simulink model "SG__DMA_test"  (R2022b)
settings: Solver=FixedStepAuto  StartTime=0.0  StopTime=2  FixedStep=50e-6  RelTol=1e-3  EnableMultiTasking=on
undefined symbols (not defined in the file or in its folder): Ended, Single
libraries: speedgoatlib_IO104 x3, speedgoatlib_IO135 x3, dspsrcs4 x2, speedgoatlib_interrupt x1
Description:
  | IO135 - DMA Loopback
settings Model: sg_rtwmakecfg_data=_sglibc_  ModifiedByFormat=Speedgoat  SimulationMode=external  PauseTimes=0  ExtModeTrigDuration=100000  Creator=Speedgoat  LastModifiedBy=Speedgoat
settings SolverCC: ConcurrentTasks=on  AlgebraicLoopSolver=TrustRegion  PositivePriorityOrder=on  AutoInsertRateTranBlk=on  InsertRTBMode=Never (minimum delay)
settings DataIOCC: SaveFormat=StructureWithTime  ReturnWorkspaceOutputs=off
settings OptimizationCC: BlockReduction=off  OptimizeBlockIOStorage=off  BufferReuse=off  ReuseModelBlockBuffer=on  GlobalBufferReuse=off  ExpressionFolding=off  LocalBlockOutputs=off
settings DebuggingCC: TasksWithSamePriorityMsg=none  UnconnectedInputMsg=warning  UnconnectedOutputMsg=warning  UnconnectedLineMsg=warning  SFExecutionAtInitializationDiag=none  ArithmeticOperatorsInVariantConditions=warning
settings HardwareCC: ProdBitPerLong=64  ProdLongLongMode=on  ProdHWDeviceType=Intel->x86-64 (Linux 64)
settings ModelReferenceCC: EnableRefExpFcnMdlSchedulingChecks=on
settings SFSimCC: SimUseLocalCustomCode=off  CustomCodeUndefinedFunction=UseInterfaceOnly
settings RTWCC: Description=Simulink Real-Time  SystemTargetFile=slrealtime.tlc  TemplateMakefile=slrealtime_default_tmf  PostCodeGenCommand=sg.model.build.makeCfg(bdroot, buildInfo);  RTWUseLocalCustomCode=off  Toolchain=Simulink Real-Time Toolchain  BuildConfiguration=Faster Runs  CodeExecutionProfiling=on  TargetLang=C++  DLArmComputeVersion=19.05
settings CodeAppCC: StateflowObjectComments=on
settings SimulinkRealTimeTargetCC: SLRTFileLogMaxRuns=10  UseGCCFastMath=on

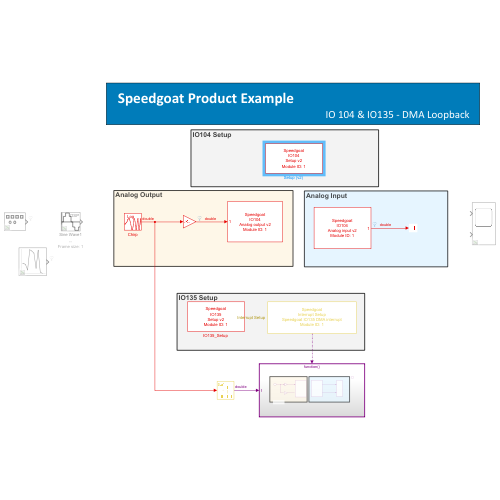
[thumbnail: Simulink's stored preview of the top-level diagram]
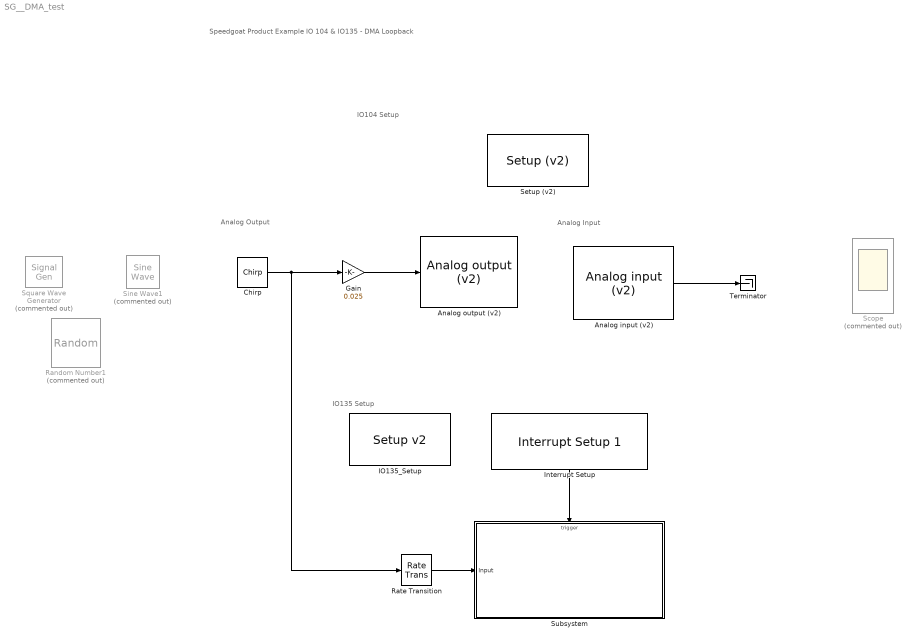
== system SG__DMA_test ==
  note: IO104 Setup
  note: Speedgoat Product Example
      | IO 104 & IO135 - DMA Loopback
  note: IO135 Setup
  note: Analog Output
  note: Analog Input
  "Analog input (v2) " : speedgoatlib_IO104/Analog input (v2)   parModuleId=1  parTs=50e-6  parPciSlot=-1  parAdChannels=1  parAdChannelsSorted=1  parAdRange1=+-5V  parAdRange2=+-5V  parAdCoupling=Single-Ended  parAdFrameSize=1  parAdUseTrigger=off  parAdClockInitiator=Initiator  parAdSampleTime=3.499503968e-05  parTriggerInitiator=Initiator  parTriggerRate=-1.000000000e+00
      settings: SourceProductName=Simulink Real-Time: Speedgoat I/O Blockset
  "Analog output (v2) " : speedgoatlib_IO104/Analog output (v2)   parModuleId=1  parTs=50e-6  parPciSlot=-1  parDaSimultaneous=on  parDaChannels=1  parDaChannelsSorted=1  parDaInitValue=0  parDaReset=1  parDaRange=+-5V  parDaFrameSize=1  parDaUseTrigger=off  parDaClockInitiator=Initiator  parDaSampleTime=3.499503968e-05  parTriggerInitiator=Initiator  parTriggerRate=-1.000000000e+00  parAdBlockPresent=1
      settings: SourceProductName=Simulink Real-Time: Speedgoat I/O Blockset
  Chirp : dspsrcs4/Chirp  sweep=Logarithmic  mode=Unidirectional  f0=1  f1=1000  t1=2  Tsweep=2  phase=0  Ts=50e-6  spf=1  datatype=Double  OutputFrames=off
  Gain : Gain  Gain=0.025
  "IO135_Setup " : speedgoatlib_IO135/Setup v2   parPciSlot=-1  parModuleId=1  parInterModuleSync=None  parConvClockBaseRate=20MHz  parConvClock1Divider=700  parConvClock2Divider=700  parFrameTriggerEnable=off  parFrameTriggerDivider=10  parConvClock1BaseRate=1  parConvClock2BaseRate=1  parFrameTriggerClock=1  parAdcChannels=[1:2]  parAdcRange1=+-10V  parAdcRange2=+-10V  parAdcRange3=+-10V  parAdcRange4=+-10V  parAdcVoltageRange=[2 2 2 2]  parAdcOversampling1=None  parAdcOversampling2=None  parAdcOversampling3=None  parAdcOversampling4=None  parAdcOversamplRate=[1 1 1 1]  parAdcAutoCorrection=on  parAdcContSampling=off  parAdcDmaEnable=on  parAdcDmaClock=Clock 1  parAdcFrameSize_=1  parAdcSampleTime_=-1  parAdcActiveDmaDevices=[1 1 1 1]  parAdcFrameTriggerEnable=0  parAdcFrameSize=1  parAdcSampleTime=3.5e-05  parDacChannels=[1:2]  parDacInitValues=0  parDacReset=1  parDacRange1=+-10V  parDacRange2=+-10V  parDacRange3=+-10V  parDacRange4=+-10V  parDacRange5=+-10V  parDacRange6=+-10V  parDacRange7=+-10V  parDacRange8=+-10V  parDacRange9=+-10V  parDacRange10=+-10V  parDacRange11=+-10V  parDacRange12=+-10V  parDacRange13=+-10V  parDacRange14=+-10V  parDacRange15=+-10V  parDacRange16=+-10V  parDacVoltageRange=[5 5 5 5 5 5 5 5 5 5 5 5 5 5 5 5]  parDacAutoCorrection=on  parDacSyncOut=on  parDacDmaEnable=on  parDacDmaLatency=Until next frame  parDacDmaClock=Clock 1  parDacFrameSize_=1  parDacSampleTime_=-1  parDacActiveDmaDevices=[1 1 1 1]  parDacFrameTriggerEnable=0  parDacFrameSize=1  parDacSampleTime=3.5e-05  parDoChannels=1  parDoInitValues=0  parDoReset=1  parDiChannels=5  parDiDebounceEnable=off  parDiDebounceTime=0  parDiDebounceValue=0  parDioPullRefFront=Pull-up 3.3V  parDioPullRefRear=Floating
      settings: SourceProductName=Simulink Real-Time: Speedgoat I/O Blockset
  Interrupt Setup : speedgoatlib_interrupt/Interrupt Setup 1  parModuleTrigger=off  parPollingMode=off  parPriorityConf=High  parPriority=254  confStartFcn=IO135_start_public  confStopFcn=IO135_stop_public  confIsrFcn=IO135_isr_public  confMapFcn=IO135_map_public  confHookFile=io135_int_hooks.c  confIrqNr=-1  confIsMdlTrig=off  confIsPolling=off  confPriority=254  confModID=16776961  confSelectedInt=Speedgoat IO135 DMA interrupt  confSelectedId=1  confSelectedChannel=[]
  Random Number1 : RandomNumber  Commented=on  SampleTime=35e-6
  Rate Transition : RateTransition  Deterministic=off
  Scope : Scope  Commented=on  NumInputPorts=2
  "Setup (v2) " : speedgoatlib_IO104/Setup (v2)   parPciSlot=-1  parModuleId=1  parTriggerInitiator=Initiator  parTriggerRate=3.499503968e-05  parCalibrate=off  parAdChannels=[1]  parAdRange1=+-5V  parAdRange2=+-5V  parAdCoupling=Single-Ended  parAdUseTrigger=off  parAdFrameSize=1  parAdClockInitiator=Initiator  parAdSampleTime=3.499503968e-05  parDaSimultaneous=on  parDaChannels=[1]  parDaChannelsSorted=1  parDaInitValue=[0]  parDaReset=[1]  parDaRange=+-5V  parDaUseTrigger=off  parDaFrameSize=1  parDaClockInitiator=Initiator  parDaSampleTime=3.499503968e-05  parDioByte0Dir=Outputs  parDioByte1Dir=Inputs  parDoChannels=[1:4]  parDoInitValues=[0]  parDoReset=[1]  parDiChannels=[13:16]
      settings: SourceProductName=Simulink Real-Time: Speedgoat I/O Blockset
  Sine Wave1 : dspsrcs4/Sine Wave  Commented=on  Amplitude=1  Frequency=500  Phase=0  SampleMode=Discrete  OutComplex=Real  CompMethod=Trigonometric fcn  TableSize=Speed  SampleTime=35e-6  SamplesPerFrame=1  ResetState=Restart at time zero  OutputFrames=off  dataType=double  wordLen=16  udDataType=sfix(16)  fracBitsMode=Best precision  numFracBits=15  OutDataTypeStr=double  LastOutDataTypeStr=double
      settings: AttributesFormatString=|
      | --
      | Frame size: %<SamplesPerFrame>
  Square Wave Generator : SignalGenerator  Commented=on  WaveForm=square  Frequency=1000
  Subsystem : Subsystem
  Terminator : Terminator
  wires:
  Interrupt Setup/1 -> Subsystem/Trigger
  Rate Transition/1 -> Subsystem/1(Input)
  "Analog input (v2) "/1 -> Terminator/1
  Chirp/1 -> Rate Transition/1, Gain/1
  Gain/1 -> "Analog output (v2) "/1

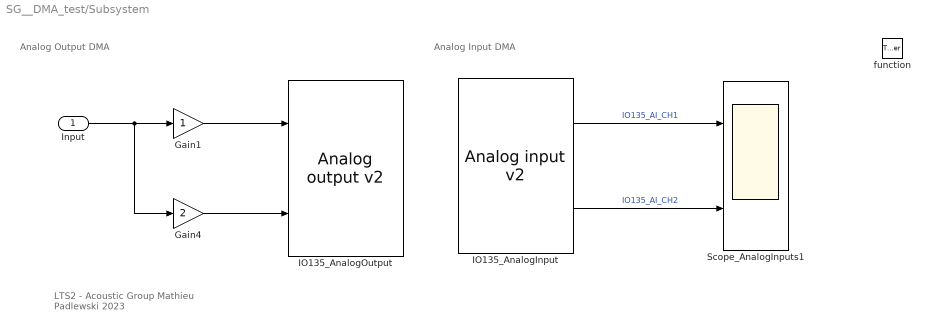
== system SG__DMA_test/Subsystem ==
  note: LTS2 - Acoustic Group
      | Mathieu Padlewski
      | 2023
  note: Analog Output DMA
  note: Analog Input DMA
  Input : Inport
  function : TriggerPort  TriggerType=function-call  VariantControl=(inherit)
  Gain1 : Gain
  Gain4 : Gain  Gain=2
  "IO135_AnalogInput " : speedgoatlib_IO135/Analog input v2   parModuleId=1  parSampleTime=-1  parPciSlot=-1  parAdcChannels=[1 2]  parAdcVoltageRange=[2 2 2 2]  parAdcOversamplRate=[1 1 1 1]  parAdcContSampling=0  parAdcDmaEnable=1  parAdcActiveDmaDevices=[1 1 1 1]  parAdcFrameSize=1
      settings: SourceProductName=Simulink Real-Time: Speedgoat I/O Blockset
  "IO135_AnalogOutput " : speedgoatlib_IO135/Analog output v2   parModuleId=1  parSampleTime=-1  parPciSlot=-1  parDacChannels=[1 2]  parDacVoltageRange=[5 5 5 5 5 5 5 5 5 5 5 5 5 5 5 5]  parDacInitValues=[0 0]  parDacReset=[1 1]  parDacSyncOut=1  parDacDmaEnable=1  parDacActiveDmaDevices=[1 1 1 1]  parDacDmaLatency=2  parDacFrameSize=1
      settings: SourceProductName=Simulink Real-Time: Speedgoat I/O Blockset
  Scope_AnalogInputs1 : Scope  NumInputPorts=2
      settings: AttributesFormatString=|
      | ---
      | %<FrameBasedProcessingString>
  wires:
  Gain4/1 -> "IO135_AnalogOutput "/2
  "IO135_AnalogInput "/1 -> Scope_AnalogInputs1/1  "IO135_AI_CH1"
  Input/1 -> Gain1/1, Gain4/1
  "IO135_AnalogInput "/2 -> Scope_AnalogInputs1/2  "IO135_AI_CH2"
  Gain1/1 -> "IO135_AnalogOutput "/1
